simulink model "ex4p2"  (R2016b)
settings: Solver=VariableStepAuto  StartTime=0.0  StopTime=0.2  RelTol=1e-3
InitFcn:
  | alpha = 60;
libraries: powerlib x9, powerlib_meascontrol x4, simulink x4
settings Model: Creator=user  LastModifiedBy=user

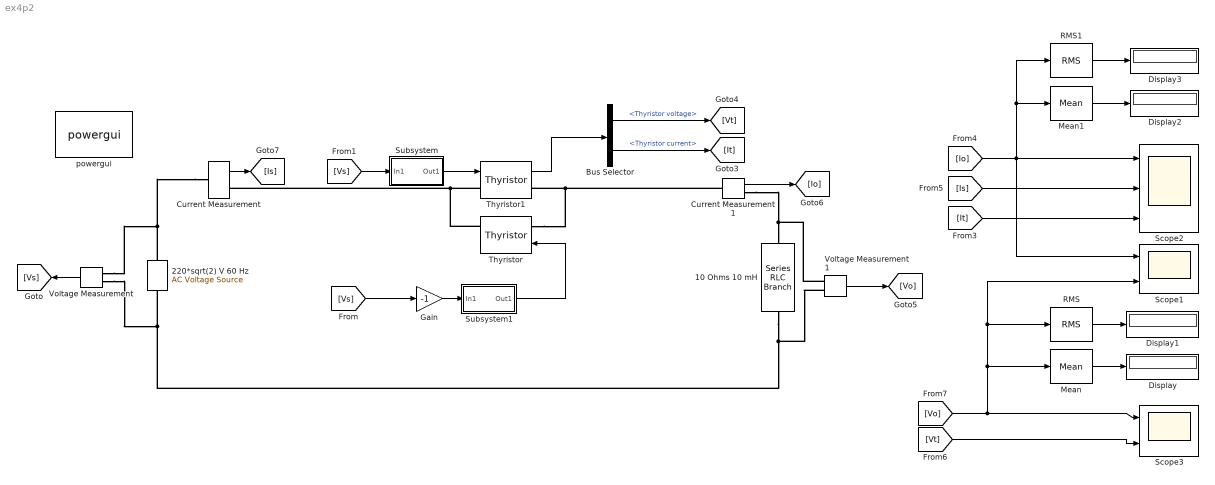
== system ex4p2 ==
  "10 Ohms 10 mH " : powerlib/Elements/Series RLC Branch  LConnTagsString=__new0  RConnTagsString=__new0  BranchType=RL  Resistance=10  Inductance=10e-3  SetiL0=off  InitialCurrent=0  Capacitance=1e-6  Setx0=off  InitialVoltage=0  Measurements=None
  220*sqrt(2) V 60 Hz : powerlib/Electrical Sources/AC Voltage Source  Amplitude=220*sqrt(2)  Phase=0  Frequency=60  SampleTime=0  Measurements=None  BusType=swing  Pref=10e3  Qref=0  Qmin=-inf  Qmax=+inf
  Bus Selector : BusSelector  OutputSignals=Thyristor voltage,Thyristor current
  Current Measurement : powerlib/Measurements/Current Measurement  PhasorSimulation=off  OutputType=Complex  PSBequivalent=0
  Current Measurement1 : powerlib/Measurements/Current Measurement  PhasorSimulation=off  OutputType=Complex  PSBequivalent=0
  Display{,1..3} (4 alike) : Display
  Gain : Gain  Gain=-1
  Mean : powerlib_meascontrol/Measurements/Mean  Freq=60  Vinit=0  Ts=0
  Mean1 : powerlib_meascontrol/Measurements/Mean  Freq=60  Vinit=0  Ts=0
  RMS : powerlib_meascontrol/Measurements/RMS  TrueRMS=on  Freq=60  RMSInit=120  Ts=0
  RMS1 : powerlib_meascontrol/Measurements/RMS  TrueRMS=on  Freq=60  RMSInit=120  Ts=0
  Scope1 : Scope  NumInputPorts=2
  Scope2 : Scope  NumInputPorts=3
  Scope3 : Scope  NumInputPorts=2
  Subsystem : Subsystem
  Subsystem1 : Subsystem
  Thyristor : powerlib/Power Electronics/Thyristor  Ron=0.001  Lon=0  Vf=0.8  IC=0  Rs=500  Cs=250e-9  Measurements=on
  Thyristor1 : powerlib/Power Electronics/Thyristor  Ron=0.001  Lon=0  Vf=0.8  IC=0  Rs=500  Cs=250e-9  Measurements=on
  Voltage Measurement : powerlib/Measurements/Voltage Measurement  PhasorSimulation=off  OutputType=Complex  PSBequivalent=0
  Voltage Measurement1 : powerlib/Measurements/Voltage Measurement  PhasorSimulation=off  OutputType=Complex  PSBequivalent=0
  powergui : powerlib/powergui  Priority=1  SimulationMode=Continuous  SolverType=Tustin/Backward Euler (TBE)  SampleTime=50e-6  frequency=60  SPID=off  DisableSnubberDevices=off  DisableRonSwitches=off  DisableVfSwitches=off  SwTol=0  DisplayEquations=off  Interpol=off  ExternalGateDelay=off  methode=off  Ts=10  FunctionMessages=off  echomessages=off  HookPort=off  EnableUseOfTLC=off  x0status=blocks  frequencyindice=60  Pbase=100e6  ErrMax=1e-4  Iterations=50  UnitsV=kV  UnitsW=MW  buscounter=0  RestoreLinks=warning  ResistiveCurrentMeasurement=off  Frange=[0:2:500]  Ylog=off  Xlog=on  ShowGrid=off  save=off  variable=ZData  structure=0  ZoomFFT=off  StartTime=0.0  cycles=1  DisplayStyle=1  fundamental=60  FreqAxis=off  MaxFrequency=1000  frequencyindicesteady=1  RmsSteady=1  display=off
  wires:
  Thyristor1/1 -> Bus Selector/1
  Voltage Measurement/1 -> [Vs]
  Current Measurement/1 -> [Is]
  Current Measurement1/1 -> [Io]
  Voltage Measurement1/1 -> [Vo]
  Bus Selector/1 -> [Vt]  "<Thyristor voltage>"
  Bus Selector/2 -> [It]  "<Thyristor current>"
  RMS1/1 -> Display3/1
  Mean1/1 -> Display2/1
  RMS/1 -> Display1/1
  Mean/1 -> Display/1
  [Io] -> Scope1/1, Mean1/1, RMS1/1, Scope2/1
  [Is] -> Scope2/2
  [It] -> Scope2/3
  [Vo] -> Mean/1, RMS/1, Scope1/2, Scope3/1
  [Vt] -> Scope3/2
  Subsystem/1(Out1) -> Thyristor1/1
  [Vs] -> Subsystem/1(In1)
  [Vs] -> Gain/1
  Gain/1 -> Subsystem1/1(In1)
  Subsystem1/1(Out1) -> Thyristor/1
  connections:
  Current Measurement/LConn1 -- 220*sqrt(2) V 60 Hz/RConn1 -- Voltage Measurement/LConn1
  Thyristor1/LConn1 -- Thyristor/RConn1 -- Current Measurement/RConn1
  Thyristor1/RConn1 -- Thyristor/LConn1 -- Current Measurement1/LConn1
  Current Measurement1/RConn1 -- "10 Ohms 10 mH "/LConn1 -- Voltage Measurement1/LConn1
  Voltage Measurement/LConn2 -- 220*sqrt(2) V 60 Hz/LConn1 -- "10 Ohms 10 mH "/RConn1 -- Voltage Measurement1/LConn2

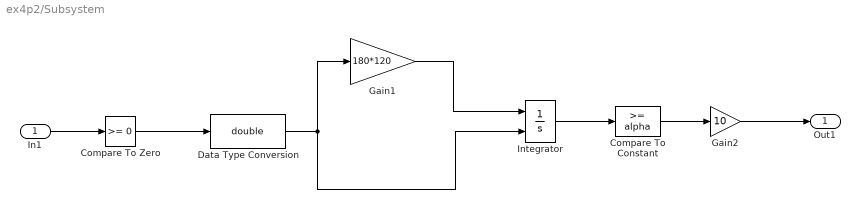
== system ex4p2/Subsystem ==
  In1 : Inport
  Compare To Constant : simulink/Logic and Bit Operations/Compare To Constant  relop=>=  const=alpha  OutDataTypeStr=boolean
  Compare To Zero : simulink/Logic and Bit Operations/Compare To Zero  relop=>=  OutDataTypeStr=boolean
  Data Type Conversion : DataTypeConversion  OutDataTypeStr=double
  Gain1 : Gain  Gain=180*120
  Gain2 : Gain  Gain=10
  Integrator : Integrator  ExternalReset=falling
  Out1 : Outport
  wires:
  Compare To Zero/1 -> Data Type Conversion/1
  Gain1/1 -> Integrator/1
  Data Type Conversion/1 -> Gain1/1, Integrator/2
  Integrator/1 -> Compare To Constant/1
  Gain2/1 -> Out1/1
  In1/1 -> Compare To Zero/1
  Compare To Constant/1 -> Gain2/1

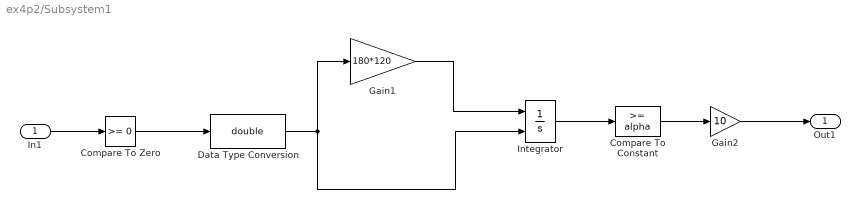
== system ex4p2/Subsystem1 ==
  In1 : Inport
  Compare To Constant : simulink/Logic and Bit Operations/Compare To Constant  relop=>=  const=alpha  OutDataTypeStr=boolean
  Compare To Zero : simulink/Logic and Bit Operations/Compare To Zero  relop=>=  OutDataTypeStr=boolean
  Data Type Conversion : DataTypeConversion  OutDataTypeStr=double
  Gain1 : Gain  Gain=180*120
  Gain2 : Gain  Gain=10
  Integrator : Integrator  ExternalReset=falling
  Out1 : Outport
  wires:
  Compare To Zero/1 -> Data Type Conversion/1
  Gain1/1 -> Integrator/1
  Data Type Conversion/1 -> Gain1/1, Integrator/2
  Integrator/1 -> Compare To Constant/1
  Gain2/1 -> Out1/1
  In1/1 -> Compare To Zero/1
  Compare To Constant/1 -> Gain2/1
